simulink model "filter_model"  (R2020b)
settings: Solver=VariableStepAuto  StartTime=0.0  StopTime=t_stop  RelTol=1e-3
values from neighbouring files (symbols this model uses):
  alpha = den_ts    [IIR_delta_filter_sim.m]
  beta = num_ts    [IIR_delta_filter_sim.m]
  ts = 1/fs    (= 8.85770975057e-08)    [IIR_delta_filter_sim.m]
undefined symbols (not defined in the file or in its folder): k
settings Model: Creator=Legion  LastModifiedBy=joseph

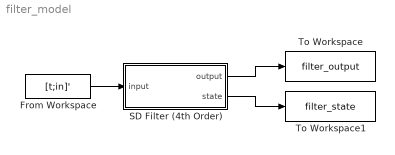
== system filter_model ==
  From Workspace : FromWorkspace  VariableName=[t;in]'  SampleTime=ts
  SD Filter (4th Order) : Subsystem
  To Workspace : ToWorkspace  VariableName=filter_output  SaveFormat=Structure With Time  SampleTime=-1
  To Workspace1 : ToWorkspace  VariableName=filter_state  SaveFormat=Structure With Time  SampleTime=-1
  wires:
  From Workspace/1 -> SD Filter (4th Order)/1(input)
  SD Filter (4th Order)/1(output) -> To Workspace/1
  SD Filter (4th Order)/2(state) -> To Workspace1/1

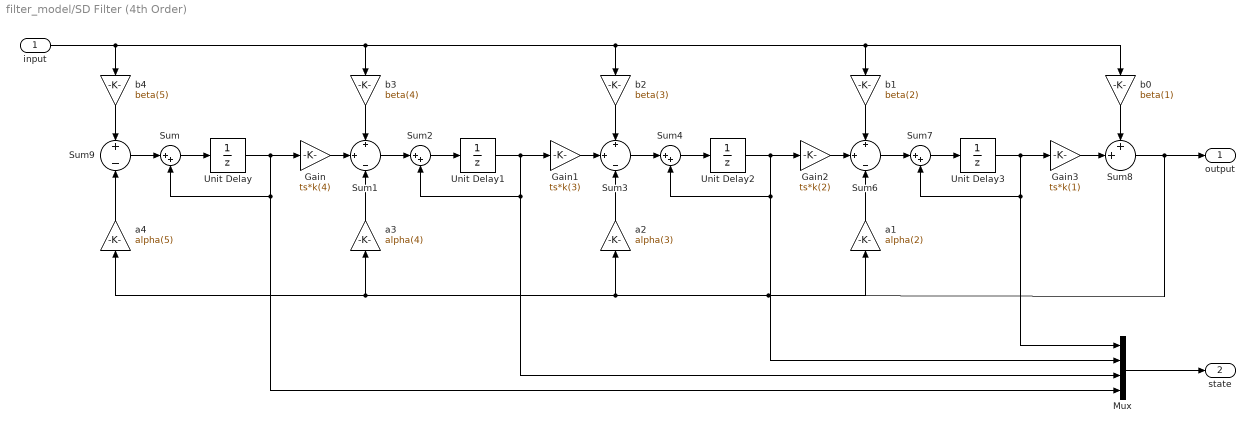
== system filter_model/SD Filter (4th Order) ==
  input : Inport
  Gain : Gain  Gain=ts*k(4)  RndMeth=Round
  Gain1 : Gain  Gain=ts*k(3)  RndMeth=Round
  Gain2 : Gain  Gain=ts*k(2)  RndMeth=Round
  Gain3 : Gain  Gain=ts*k(1)  RndMeth=Round
  Mux : Mux
  Sum{,2,4,7} (4 alike) : Sum  Inputs=|++
  Sum1 : Sum  Inputs=+|+|-
  Sum3 : Sum  Inputs=+|+|-
  Sum6 : Sum  Inputs=+|+|-
  Sum8 : Sum  Inputs=++|
  Sum9 : Sum  Inputs=+|-
  Unit Delay{,1..3} (4 alike) : UnitDelay  SampleTime=-1  HasFrameUpgradeWarning=on
  a1 : Gain  Gain=alpha(2)
  a2 : Gain  Gain=alpha(3)
  a3 : Gain  Gain=alpha(4)
  a4 : Gain  Gain=alpha(5)
  b0 : Gain  Gain=beta(1)
  b1 : Gain  Gain=beta(2)
  b2 : Gain  Gain=beta(3)
  b3 : Gain  Gain=beta(4)
  b4 : Gain  Gain=beta(5)
  output : Outport
  state : Outport  Port=2
  wires:
  a1/1 -> Sum6/3
  Sum9/1 -> Sum/1
  b0/1 -> Sum8/1
  Sum6/1 -> Sum7/1
  a4/1 -> Sum9/2
  b3/1 -> Sum1/1
  Unit Delay3/1 -> Mux/1, Sum7/2, Gain3/1
  b1/1 -> Sum6/1
  Gain/1 -> Sum1/2
  Unit Delay1/1 -> Mux/3, Sum2/2, Gain1/1
  Sum3/1 -> Sum4/1
  input/1 -> b0/1, b1/1, b2/1, b3/1, b4/1
  Gain2/1 -> Sum6/2
  b2/1 -> Sum3/1
  Unit Delay2/1 -> Mux/2, Sum4/2, Gain2/1
  Gain1/1 -> Sum3/2
  Sum1/1 -> Sum2/1
  a2/1 -> Sum3/3
  Gain3/1 -> Sum8/2
  b4/1 -> Sum9/1
  Sum/1 -> Unit Delay/1
  Sum4/1 -> Unit Delay2/1
  Sum7/1 -> Unit Delay3/1
  Sum2/1 -> Unit Delay1/1
  a3/1 -> Sum1/3
  Unit Delay/1 -> Mux/4, Sum/2, Gain/1
  Sum8/1 -> output/1, a4/1, a3/1, a2/1, a1/1
  Mux/1 -> state/1
